simulink model "Ball_and_Beam"  (R2018a)
settings: Solver=VariableStepAuto  StartTime=0.0  StopTime=600  RelTol=1e-3
settings Model: Creator=Zeljko  LastModifiedBy=Zeljko

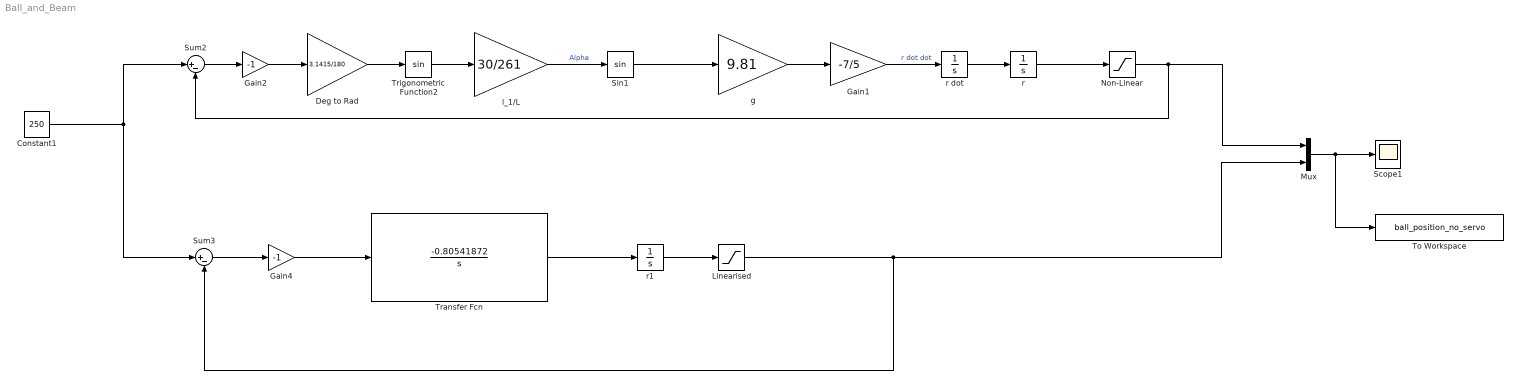
== system Ball_and_Beam ==
  Constant1 : Constant  Value=250
  Deg to Rad : Gain  Gain=3.1415/180
  Gain1 : Gain  Gain=-7/5
  Gain2 : Gain  Gain=-1
  Gain4 : Gain  Gain=-1
  Linearised : Saturate  UpperLimit=400  LowerLimit=0
  Mux : Mux  Inputs=2
  Non-Linear : Saturate  UpperLimit=400  LowerLimit=0
  Scope1 : Scope
  Sin1 : Trigonometry
  Sum2 : Sum  Inputs=|+-
  Sum3 : Sum  Inputs=|+-
  To Workspace : ToWorkspace  VariableName=ball_position_no_servo  SaveFormat=Timeseries  SampleTime=-1
  Transfer Fcn : TransferFcn  Numerator=[-0.80541872]  Denominator=[1 0]
  Trigonometric Function2 : Trigonometry
  g : Gain  Gain=9.81
  l_1/L : Gain  Gain=30/261
  r : Integrator  InitialCondition=100
  r dot : Integrator
  r1 : Integrator  InitialCondition=100
  wires:
  Mux/1 -> To Workspace/1, Scope1/1
  Non-Linear/1 -> Sum2/2, Mux/1
  Constant1/1 -> Sum3/1, Sum2/1
  Sum3/1 -> Gain4/1
  Gain4/1 -> Transfer Fcn/1
  Linearised/1 -> Sum3/2, Mux/2
  r1/1 -> Linearised/1
  Transfer Fcn/1 -> r1/1
  r/1 -> Non-Linear/1
  Gain1/1 -> r dot/1  "r dot dot"
  Deg to Rad/1 -> Trigonometric Function2/1
  r dot/1 -> r/1
  Sin1/1 -> g/1
  l_1/L/1 -> Sin1/1  "Alpha"
  g/1 -> Gain1/1
  Trigonometric Function2/1 -> l_1/L/1
  Sum2/1 -> Gain2/1
  Gain2/1 -> Deg to Rad/1
